simulink model "dmass_sim_sol"  (R2023b)
settings: Solver=ode3  StartTime=0.0  StopTime=H  FixedStep=0.01  RelTol=1e-3
values from neighbouring files (symbols this model uses):
  a_vect = [ k ; d ; m ]    [MSD_par_sol.m]    (also in balloon_par_sol.m = -At(3,:)'; dmass_par_sol.m = -At(4,1:4)')
  alpha_vect = poly3traj([p0;v0],[pT;vT],H)    [MSD_par_sol.m]    (also in balloon_par_sol.m = poly5traj([h0;v0;a0],[hT;vT;aT],T); dmass_par_sol.m = poly7traj(z0,zT,H))
  k = 5    [MSD_par_sol.m]    (also in dmass_par_sol.m)
  m1 = 10    [dmass_par_sol.m]
  m2 = 20    [dmass_par_sol.m]
settings Model: Creator=jerome  LastModifiedBy=jerome
settings ModelReferenceCC: EnableRefExpFcnMdlSchedulingChecks=on

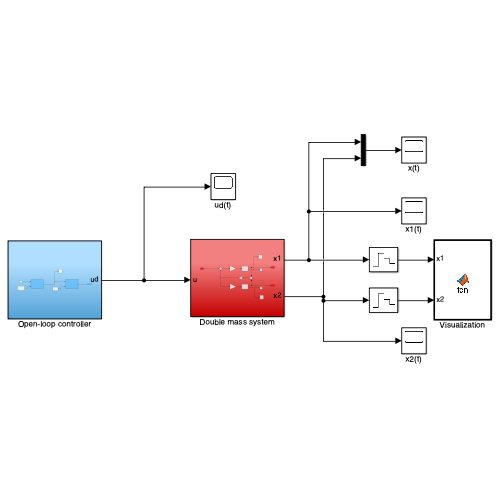
[thumbnail: Simulink's stored preview of the top-level diagram]
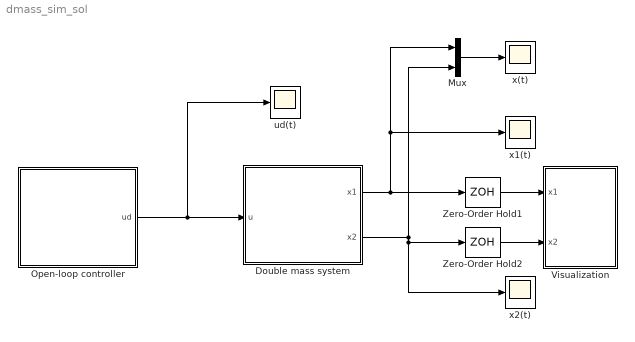
== system dmass_sim_sol ==
  Double mass system : Subsystem
  Mux : Mux  Inputs=2
  Open-loop controller : Subsystem
  Visualization : MATLAB Function  TreatAsAtomicUnit=on
  Zero-Order Hold1 : ZeroOrderHold  SampleTime=0.2
  Zero-Order Hold2 : ZeroOrderHold  SampleTime=0.2
  ud(t) : Scope
  x(t) : Scope
  x1(t) : Scope
  x2(t) : Scope
  wires:
  Open-loop controller/1(ud) -> ud(t)/1, Double mass system/1(u)
  Mux/1 -> x(t)/1
  Double mass system/1(x1) -> Zero-Order Hold1/1, Mux/1, x1(t)/1
  Zero-Order Hold2/1 -> Visualization/2(x2)
  Double mass system/2(x2) -> Mux/2, Zero-Order Hold2/1, x2(t)/1
  Zero-Order Hold1/1 -> Visualization/1(x1)

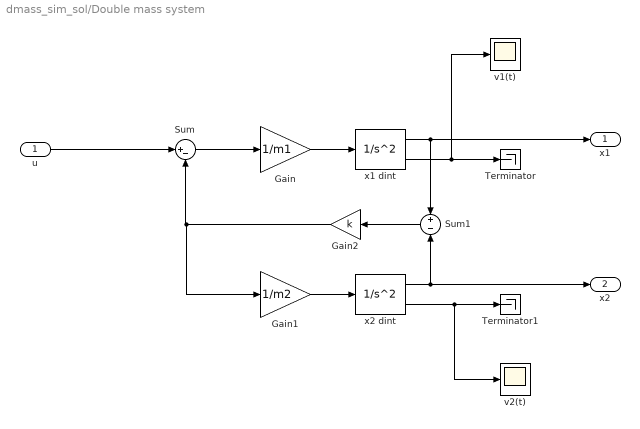
== system dmass_sim_sol/Double mass system ==
  u : Inport
  Gain : Gain  Gain=1/m1
  Gain1 : Gain  Gain=1/m2
  Gain2 : Gain  Gain=k
  Sum : Sum  Inputs=|+-
  Sum1 : Sum  Inputs=+-
  Terminator : Terminator
  Terminator1 : Terminator
  v1(t) : Scope
  v2(t) : Scope
  x1 dint : SecondOrderIntegrator  ICX=0
  x2 dint : SecondOrderIntegrator
  x1 : Outport
  x2 : Outport  Port=2
  wires:
  Sum1/1 -> Gain2/1
  x2 dint/2 -> v2(t)/1, Terminator1/1
  u/1 -> Sum/1
  x2 dint/1 -> x2/1, Sum1/2
  x1 dint/2 -> v1(t)/1, Terminator/1
  Gain/1 -> x1 dint/1
  Gain2/1 -> Sum/2, Gain1/1
  Gain1/1 -> x2 dint/1
  x1 dint/1 -> x1/1, Sum1/1
  Sum/1 -> Gain/1

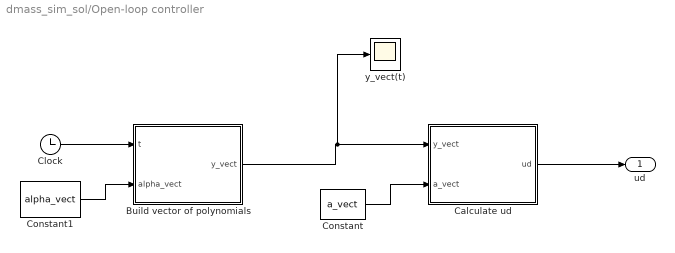
== system dmass_sim_sol/Open-loop controller ==
  Build vector of polynomials : MATLAB Function  TreatAsAtomicUnit=on
  Calculate ud : MATLAB Function  TreatAsAtomicUnit=on
  Clock : Clock
  Constant : Constant  Value=a_vect  VectorParams1D=off
  Constant1 : Constant  Value=alpha_vect  VectorParams1D=off
  y_vect(t) : Scope
  ud : Outport
  wires:
  Calculate ud/1(ud) -> ud/1
  Build vector of polynomials/1(y_vect) -> y_vect(t)/1, Calculate ud/1(y_vect)
  Constant/1 -> Calculate ud/2(a_vect)
  Constant1/1 -> Build vector of polynomials/2(alpha_vect)
  Clock/1 -> Build vector of polynomials/1(t)

== matlab function dmass_sim_sol/Open-loop controller/Calculate ud ==
  data: y_vect input; ud output; a_vect input
function ud = fcn(y_vect,a_vect)

ae_vect = [ a_vect ; 1 ]; % extended parameter vector

ud = ae_vect' * y_vect;

== matlab function dmass_sim_sol/Visualization ==
  data: x1 input; x2 input
function fcn(x1,x2)


so = 12; % spring offset
% mass 1
    Xmass1 = [ 5 ; 5 ; -5 ; -5 ; 5 ] + x1 - so;
    Ymass1 = [ -5 ; 5 ; 5 ; -5 ; -5]; 

% mass 2
    Xmass2 = [ 5 ; 5 ; -5 ; -5 ; 5 ] + x2 + so;
    Ymass2 = [ -5 ; 5 ; 5 ; -5 ; -5]; 

% the spring
    Xspring = [ 0 ; 4 ; 6 ; 10 ; 14 ; 18 ; 20 ; 24 ]/24*(x2-x1+2*so-10) + (x1-so+5);
    Yspring = [ 0 ; 0 ; 3 ; -3 ; 3 ; -3 ; 0 ; 0 ];

% to be able to use 'fill' even though the function is not supported for code generation
% see https://se.mathworks.com/help/simulink/slref/coder.extrinsic.html
coder.extrinsic('fill'); 

% draw the masses
fill(Xmass1,Ymass1,'r');
hold on
fill(Xmass2,Ymass2,'r');

% draw the spring
plot(Xspring,Yspring,'b','Linewidth',3);

% draw misc
plot([-so -so],[-10 -7],'k','Linewidth',2);  %draw a thin line at position x1 = 0
plot([so so],[-10 -7],'k','Linewidth',2);  %draw a thin line at position x2 = 0
hold off

axis([-20 60 -10 10]);
title('Mass-Spring-Damper system', 'FontSize',20);
axis equal;
grid on;

drawnow;

== matlab function dmass_sim_sol/Open-loop controller/Build vector of polynomials ==
  data: t input; y_vect output; alpha_vect input
function y_vect = fcn(t,alpha_vect)

% if poly7traj is used
t_vect0 = [ 1 ; t ; t^2 ; t^3 ; t^4 ; t^5 ; t^6 ; t^7 ];
t_vect1 = [ 0 ; 1 ; 2*t ; 3*t^2 ; 4*t^3 ; 5*t^4 ; 6*t^5 ; 7*t^6 ];
t_vect2 = [ 0 ; 0 ; 2 ; 2*3*t ; 3*4*t^2 ; 4*5*t^3 ; 5*6*t^4 ; 6*7*t^5 ];
t_vect3 = [ 0 ; 0 ; 0 ; 2*3 ; 2*3*4*t ; 3*4*5*t^2 ; 4*5*6*t^3 ; 5*6*7*t^4 ];
t_vect4 = [ 0 ; 0 ; 0 ; 0 ; 2*3*4 ; 2*3*4*5*t ; 3*4*5*6*t^2 ; 4*5*6*7*t^3 ];


yd = t_vect0'*alpha_vect;
yd_dot = t_vect1'*alpha_vect;
yd_ddot = t_vect2'*alpha_vect;
yd_3dot = t_vect3'*alpha_vect;
yd_4dot = t_vect4'*alpha_vect;

y_vect = [ yd ; yd_dot ; yd_ddot ; yd_3dot ; yd_4dot ];
